simulink model "nicht_lin1"  (Simulink 4.00)
settings: Solver=ode45  StartTime=0.0  StopTime=20.0  RelTol=1e-3
values from neighbouring files (symbols this model uses):
  Kd = 1.9688    [ident21.mat]    (also in nicht_lin1_1.mat = 3.77195826555; nicht_lin2.mat = 4.01612566605)
  Ki = 0    [ident21.mat]    (also in nicht_lin1_1.mat = 1.3829465335; nicht_lin2.mat = 1.48579685399)
  Kp = 4.81125224325    [ident21.mat]    (also in nicht_lin1_1.mat = 1.99795408441; nicht_lin2.mat = 2.13666402957)
settings Model: LastModifiedBy=Administrator  BlockReductionOpt=off

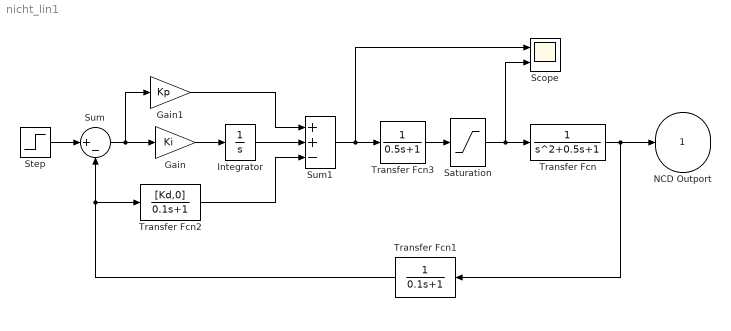
== system nicht_lin1 ==
  Gain : Gain  Gain=Ki  Multiplication=Element-wise(K.*u)  SaturateOnIntegerOverflow=on
  Gain1 : Gain  Gain=Kp  Multiplication=Element-wise(K.*u)  SaturateOnIntegerOverflow=on
  Integrator : Integrator  ExternalReset=none  InitialConditionSource=internal  InitialCondition=0  LimitOutput=off  UpperSaturationLimit=inf  LowerSaturationLimit=-inf  ShowSaturationPort=off  ShowStatePort=off  AbsoluteTolerance=auto
  Saturation : Saturate  UpperLimit=1.0  LowerLimit=-1.0  LinearizeAsGain=on
  Scope : Scope  NumInputPorts=2
      settings: TimeRange=auto  YMin=-5~-5  YMax=5~5  SaveToWorkspace=off  SaveName=ScopeData  LimitDataPoints=on  MaxDataPoints=5000
  Step : Step  Time=0  Before=0  After=1  SampleTime=0
  Sum : Sum  Inputs=|+-  SaturateOnIntegerOverflow=on
  Sum1 : Sum  Inputs=++-  SaturateOnIntegerOverflow=on
  Transfer Fcn : TransferFcn  Numerator=[1]  Denominator=[1 0.5 1]  Realization=auto  AbsoluteTolerance=auto
  Transfer Fcn1 : TransferFcn  Orientation=left  Numerator=[1]  Denominator=[0.1 1]  Realization=auto  AbsoluteTolerance=auto
  Transfer Fcn2 : TransferFcn  Numerator=[Kd,0]  Denominator=[0.1, 1]  Realization=auto  AbsoluteTolerance=auto
  Transfer Fcn3 : TransferFcn  Numerator=[1]  Denominator=[0.5 1]  Realization=auto  AbsoluteTolerance=auto
  NCD Outport : Outport  Port=1  InitialOutput=0
      settings: OpenFcn=optblock
      mask Type: NCD Outport
      mask Display:
      | plot([0:10],[-.5 1.5 .6 1.3 .8 1.1 .95 1.02 .99 1 1]);
      | disp('\n\n NCD\n OutPort 1');
  wires:
  Step/1 -> Sum/1
  Transfer Fcn/1 -> NCD Outport/1, Transfer Fcn1/1
  Transfer Fcn1/1 -> Sum/2, Transfer Fcn2/1
  Sum/1 -> Gain/1, Gain1/1
  Sum1/1 -> Scope/1, Transfer Fcn3/1
  Gain1/1 -> Sum1/1
  Gain/1 -> Integrator/1
  Transfer Fcn2/1 -> Sum1/3
  Integrator/1 -> Sum1/2
  Saturation/1 -> Transfer Fcn/1, Scope/2
  Transfer Fcn3/1 -> Saturation/1
